simulink model "ass3q1e"  (R2025a)
settings: Solver=VariableStepAuto  StartTime=0.0  StopTime=100  RelTol=1e-3
values from neighbouring files (symbols this model uses):
  D = 20 / ( 2 * pi)    (= 3.18309886184)    [assignement_3_simulink_q1.m]    (also in ecse563_part1c_model.m)
  M = length(nfrom)    [admittance.m]    (also in assignement_3_simulink_q1.m = 111.41; ecse563_part1c_model.m = 111.4; nrpf.m = zeros(nb, nb))
  R1 = 0.0060 * 2 * pi    (= 0.0376991118431)    [assignement_3_simulink_q1.m]
  R2 = 0.0120 * 2 * pi    (= 0.0753982236862)    [assignement_3_simulink_q1.m]
  Tch1 = 3    [assignement_3_simulink_q1.m]
  Tch2 = 8    [assignement_3_simulink_q1.m]
  Tg1 = 0.25    [assignement_3_simulink_q1.m]
  Tg2 = 0.50    (= 0.5)    [assignement_3_simulink_q1.m]
settings Model: Creator=aliseifeldin  LastModifiedBy=aliseifeldin

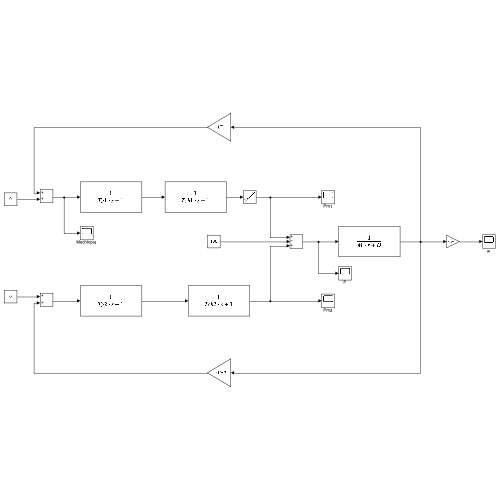
[thumbnail: Simulink's stored preview of the top-level diagram]
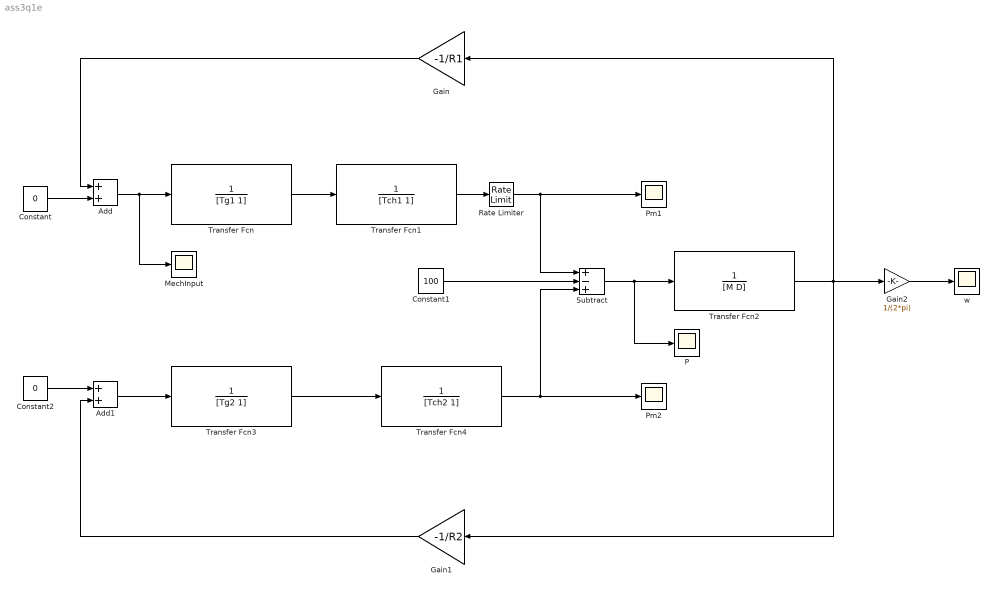
== system ass3q1e ==
  Add : Sum
  Add1 : Sum
  Constant : Constant  Value=0
  Constant1 : Constant  Value=100
  Constant2 : Constant  Value=0
  Gain : Gain  Gain=-1/R1
  Gain1 : Gain  Gain=-1/R2
  Gain2 : Gain  Gain=1/(2*pi)
  MechInput : Scope
      settings: ActiveDisplayYMinimum=-23.085657317031824  ActiveDisplayYMaximum=207.77091585328645  DataLoggingVariableName=Pm1Scope1
  P : Scope
      settings: ActiveDisplayYMinimum=-1  ActiveDisplayYMaximum=1  DataLoggingVariableName=PScope
  Pm1 : Scope
      settings: ActiveDisplayYMinimum=-7.8864618189341318  ActiveDisplayYMaximum=70.9781563704072  DataLoggingVariableName=Pm1Scope
  Pm2 : Scope
      settings: ActiveDisplayYMinimum=-1  ActiveDisplayYMaximum=1  DataLoggingVariableName=Pm2Scope
  Rate Limiter : RateLimiter  SampleTimeMode=inherited
  Subtract : Sum  Inputs=+-+
  Transfer Fcn : TransferFcn  Denominator=[Tg1 1]
  Transfer Fcn1 : TransferFcn  Denominator=[Tch1 1]
  Transfer Fcn2 : TransferFcn  Denominator=[M D]
  Transfer Fcn3 : TransferFcn  Denominator=[Tg2 1]
  Transfer Fcn4 : TransferFcn  Denominator=[Tch2 1]
  w : Scope
      settings: ActiveDisplayYMinimum=-1  ActiveDisplayYMaximum=1  DataLoggingVariableName=wScope
  wires:
  Transfer Fcn/1 -> Transfer Fcn1/1
  Subtract/1 -> P/1, Transfer Fcn2/1
  Transfer Fcn1/1 -> Rate Limiter/1
  Transfer Fcn2/1 -> Gain2/1, Gain/1, Gain1/1
  Gain/1 -> Add/1
  Add/1 -> MechInput/1, Transfer Fcn/1
  Constant/1 -> Add/2
  Constant1/1 -> Subtract/2
  Transfer Fcn3/1 -> Transfer Fcn4/1
  Add1/1 -> Transfer Fcn3/1
  Constant2/1 -> Add1/1
  Gain1/1 -> Add1/2
  Transfer Fcn4/1 -> Pm2/1, Subtract/3
  Rate Limiter/1 -> Pm1/1, Subtract/1
  Gain2/1 -> w/1
